simulink model "BBB_I2C_Read_Test_LibraryBlock"  (R2013a)
settings: Solver=FixedStepDiscrete  StartTime=0.0  StopTime=inf  RelTol=1e-3
libraries: BLACKlink x2, simulink x2
settings Model: SimulationMode=external  ExtModeTrigDuration=100  Creator=rdustinkahawita  LastModifiedBy=rdustinkahawita
settings OptimizationCC: OptimizeModelRefInitCode=on  LifeSpan=1
settings DebuggingCC: SolverPrmCheckMsg=none  StrictBusMsg=Warning
settings HardwareCC: ProdLargestAtomicInteger=Long  ProdLargestAtomicFloat=Double  ProdEndianess=LittleEndian  ProdHWDeviceType=ARM Compatible->ARM Cortex
settings RTWCC: SystemTargetFile=realtime.tlc  GenerateMakefile=off  TemplateMakefile=realtime.tmf  Description=Run on Target Hardware  RTWVerbose=off  ProcessScript=realtime_make_rtw_hook
settings STFCustomTargetCC: TargetLibSuffix=.a  GenerateSampleERTMain=on  ERTCustomFileBanners=on  SupportNonInlinedSFcns=off  SupportVariableSizeSignals=on  MATLABClassNameForMDSCustomization=Simulink.SoftwareTarget.ERTCustomization  SystemTargetFile=realtime.tlc
settings ERTTargetCC: ParMdlRefBuildCompliant=off  CompOptLevelCompliant=off  ConcurrentExecutionCompliant=off  CombineOutputUpdateFcns=off  ERTFirstTimeCompliant=off  SupportContinuousTime=on  SupportVariableSizeSignals=on  ModelStepFunctionPrototypeControlCompliant=off  CPPClassGenCompliant=off  ExtMode=on  ExtModeMexArgs='192.168.7.2' 0 17725  ERTSrcFileBannerTemplate=realtime_code_template.cgt  ERTHdrFileBannerTemplate=realtime_code_template.cgt  ERTDataSrcFileTemplate=realtime_code_template.cgt  ERTDataHdrFileTemplate=realtime_code_template.cgt  ERTCustomFileTemplate=realtime_file_process.tlc

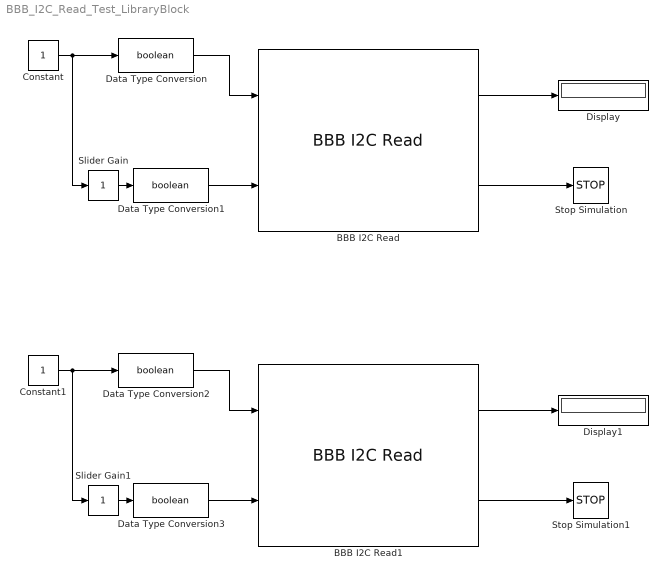
== system BBB_I2C_Read_Test_LibraryBlock ==
  BBB I2C Read : BLACKlink/BBB I2C Read  BBB_I2CBusNo=BeagleBone Black I2C Channel 1  BBB_I2CAddress=104  BBB_I2CRegister=0  BBB_DebugInfo=Debug Level 4 - Include Device Registery Read-Out
  BBB I2C Read1 : BLACKlink/BBB I2C Read  BBB_I2CBusNo=BeagleBone Black I2C Channel 1  BBB_I2CAddress=104  BBB_I2CRegister=0  BBB_DebugInfo=Debug Level 4 - Include Device Registery Read-Out
  Constant : Constant
  Constant1 : Constant
  Data Type Conversion{,1..3} (4 alike) : DataTypeConversion  OutMin=[0]  OutMax=[1]  OutDataTypeStr=boolean
  Display : Display
      settings: Format=hex (Stored Integer)
  Display1 : Display
      settings: Format=hex (Stored Integer)
  Slider Gain : simulink/Math Operations/Slider Gain  low=0  gain=1  high=1
  Slider Gain1 : simulink/Math Operations/Slider Gain  low=0  gain=1  high=1
  Stop Simulation : Stop
  Stop Simulation1 : Stop
  wires:
  Constant/1 -> Slider Gain/1, Data Type Conversion/1
  Data Type Conversion/1 -> BBB I2C Read/1
  Slider Gain/1 -> Data Type Conversion1/1
  Data Type Conversion1/1 -> BBB I2C Read/2
  BBB I2C Read/1 -> Display/1
  BBB I2C Read/2 -> Stop Simulation/1
  Constant1/1 -> Slider Gain1/1, Data Type Conversion2/1
  Data Type Conversion2/1 -> BBB I2C Read1/1
  Slider Gain1/1 -> Data Type Conversion3/1
  Data Type Conversion3/1 -> BBB I2C Read1/2
  BBB I2C Read1/1 -> Display1/1
  BBB I2C Read1/2 -> Stop Simulation1/1
